simulink model "sampleModel1642"  (R2023a)
settings: Solver=VariableStepAuto  StartTime=0.0  StopTime=10.0  RelTol=1e-3
libraries: hdlsllib x3, simulink x2
settings Model: Creator=user1  LastModifiedBy=user1

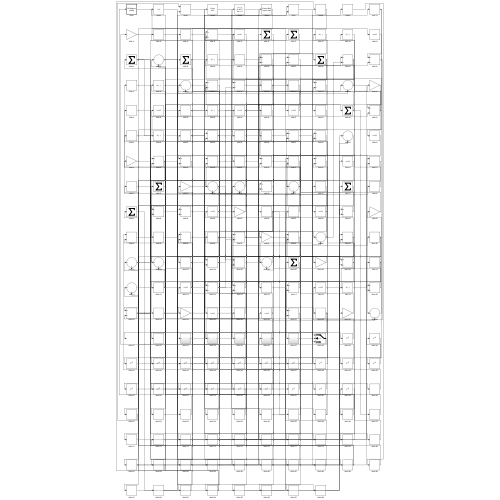
[thumbnail: Simulink's stored preview of the top-level diagram]
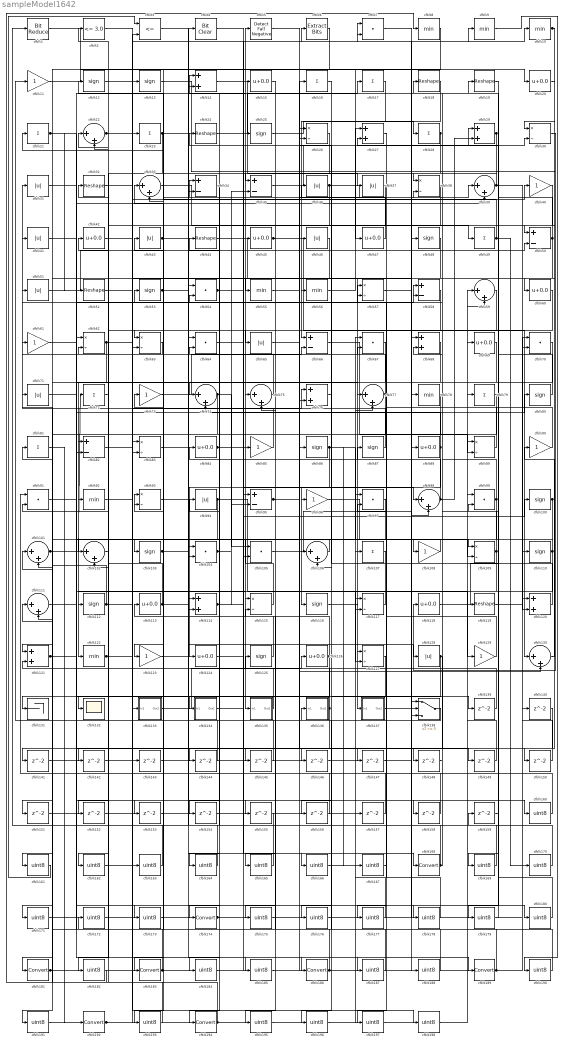
== system sampleModel1642 ==
  cfblk1 : hdlsllib/Logic and Bit Operations/Bit Reduce  mode=AND
  cfblk{8..10,55..56,78,92,122} (8 alike) : MinMax
  cfblk{12..13,25,48,53,80,86..87,100,103,110,112,116,125} (14 alike) : Signum
  cfblk{22,33,39,59,74..75,77,98,101..102,106,111,130} (13 alike) : Sum  Inputs=|++
  cfblk{7,54,64,67,70,91,97,99,104..105} (10 alike) : DotProduct  OutDataTypeStr=Inherit: Inherit via internal rule
  cfblk{16..17,21,23,28,49,72,79,81,107} (10 alike) : Sum  Inputs=+
  cfblk{11,40,61,73,85,90,96,108,123,129} (10 alike) : Gain
  cfblk{26,30,38,57,62..63,83,89,93,109,115,117,127} (13 alike) : Product  Inputs=*/  RndMeth=Zero  SaturateOnIntegerOverflow=on
  cfblk{15,20,42,45,47,60,69,84,88,113,118,124,126} (13 alike) : Bias  Bias=0.0  SaturateOnIntegerOverflow=off
  cfblk{14,27,29,68,76,114,120..121} (8 alike) : Sum
  cfblk{18..19,24,32,44,52,119} (7 alike) : Reshape
  cfblk{31,36..37,41,43,46,51,65,71,94,128} (11 alike) : Abs  SaturateOnIntegerOverflow=off
  cfblk131 : Terminator
  cfblk132 : Scope
  cfblk133 : Subsystem
      settings: LibrarySourceBlock=|
      | hdlsllib/Ports &
      | Subsystems/Subsystem
  cfblk134 : Subsystem
      settings: LibrarySourceBlock=|
      | hdlsllib/Ports &
      | Subsystems/Subsystem
  cfblk135 : Subsystem
      settings: LibrarySourceBlock=|
      | hdlsllib/Ports &
      | Subsystems/Subsystem
  cfblk136 : Subsystem
      settings: LibrarySourceBlock=|
      | hdlsllib/Ports &
      | Subsystems/Subsystem
  cfblk137 : Subsystem
      settings: LibrarySourceBlock=|
      | hdlsllib/Ports &
      | Subsystems/Subsystem
  cfblk138 : Switch  SaturateOnIntegerOverflow=off  InputSameDT=off
  cfblk{139..159} (21 alike) : Delay  SampleTime=1
  cfblk{160..167,169..173,175..180,182,184..185,187..188,190..191,193,195..198} (31 alike) : DataTypeConversion  OutDataTypeStr=uint8  SaturateOnIntegerOverflow=off  RndMeth=Floor
  cfblk{168,174,181,183,186,189,192,194} (8 alike) : DataTypeConversion  SaturateOnIntegerOverflow=off  RndMeth=Floor
  cfblk2 : hdlsllib/Logic and Bit Operations/Compare To Constant  relop=<=  const=3.0  OutDataTypeStr=boolean
  cfblk3 : RelationalOperator  Operator=<=  OutDataTypeStr=boolean  InputSameDT=off
  cfblk{34..35,50,58,66,82,95} (7 alike) : Sum  Inputs=+-
  cfblk4 : simulink/Logic and Bit Operations/Bit Clear  iBit=0
      settings: LibrarySourceBlock=|
      | hdlsllib/Logic and Bit
      | Operations/Bit Clear
  cfblk5 : hdlsllib/Logic and Bit Operations/Detect Fall Negative  vinit=0  OutDataTypeStr=boolean
  cfblk6 : simulink/Logic and Bit Operations/Extract Bits  bitsToExtract=Upper half  numBits=8  bitIdxRange=[0 7]  outScalingMode=Preserve fixed-point scaling
      settings: LibrarySourceBlock=|
      | hdlsllib/Logic and Bit
      | Operations/Extract Bits
  wires:
  cfblk68/1 -> cfblk122/1
  cfblk24/1 -> cfblk17/1
  cfblk109/1 -> cfblk51/1, cfblk193/1
  cfblk118/1 -> cfblk63/1
  cfblk11/1 -> cfblk20/1
  cfblk63/1 -> cfblk31/1
  cfblk101/1 -> cfblk72/1, cfblk80/1
  cfblk8/1 -> cfblk181/1
  cfblk13/1 -> cfblk50/1
  cfblk88/1 -> cfblk124/1, cfblk74/2
  cfblk17/1 -> cfblk66/1
  cfblk120/1 -> cfblk24/1
  cfblk5/1 -> cfblk86/1
  cfblk133/1(Out1) -> cfblk126/1
  cfblk47/1 -> cfblk12/1
  cfblk135/1(Out1) -> cfblk22/1
  cfblk45/1 -> cfblk130/1, cfblk30/2
  cfblk33/1 -> cfblk49/1
  cfblk25/1 -> cfblk28/1
  cfblk83/1 -> cfblk189/1
  cfblk28/1 -> cfblk38/1, cfblk65/1
  cfblk36/1 -> cfblk38/2, cfblk75/2
  cfblk30/1 -> cfblk118/1
  cfblk64/1 -> cfblk168/1
  cfblk82/1 -> cfblk23/1
  cfblk23/1 -> cfblk128/1, cfblk132/1
  cfblk48/1 -> cfblk137/1(In1)
  cfblk86/1 -> cfblk116/1, cfblk108/1, cfblk134/1(In1), cfblk167/1
  cfblk126/1 -> cfblk113/1, cfblk191/1
  cfblk115/1 -> cfblk5/1
  cfblk93/1 -> cfblk4/1
  cfblk14/1 -> cfblk37/1
  cfblk136/1(Out1) -> cfblk93/1, cfblk154/1
  cfblk50/1 -> cfblk14/2, cfblk27/2, cfblk195/1
  cfblk35/1 -> cfblk29/1
  cfblk100/1 -> cfblk135/1(In1), cfblk102/2
  cfblk16/1 -> cfblk96/1
  cfblk69/1 -> cfblk101/2
  cfblk116/1 -> cfblk127/1
  cfblk54/1 -> cfblk158/1, cfblk184/1
  cfblk107/1 -> cfblk174/1
  cfblk39/1 -> cfblk120/2, cfblk35/1
  cfblk81/1 -> cfblk192/1
  cfblk78/1 -> cfblk92/1
  cfblk117/1 -> cfblk114/1
  cfblk51/1 -> cfblk13/1
  cfblk134/1(Out1) -> cfblk85/1
  cfblk138/1 -> cfblk11/1
  cfblk42/1 -> cfblk40/1
  cfblk108/1 -> cfblk103/1
  cfblk77/1 -> cfblk121/1, cfblk36/1, cfblk57/2
  cfblk119/1 -> cfblk110/1
  cfblk73/1 -> cfblk66/2
  cfblk89/1 -> cfblk53/1
  cfblk18/1 -> cfblk46/1
  cfblk96/1 -> cfblk109/1
  cfblk84/1 -> cfblk14/1, cfblk7/2
  cfblk103/1 -> cfblk123/1, cfblk166/1
  cfblk53/1 -> cfblk55/1, cfblk178/1
  cfblk44/1 -> cfblk138/1
  cfblk56/1 -> cfblk27/1
  cfblk71/1 -> cfblk115/1
  cfblk66/1 -> cfblk89/2
  cfblk75/1 -> cfblk44/1
  cfblk26/1 -> cfblk183/1
  cfblk110/1 -> cfblk127/2, cfblk104/1, cfblk162/1
  cfblk92/1 -> cfblk75/1
  cfblk52/1 -> cfblk50/2
  cfblk98/1 -> cfblk84/1, cfblk29/2
  cfblk122/1 -> cfblk9/1, cfblk155/1
  cfblk4/1 -> cfblk98/1
  cfblk121/1 -> cfblk15/1, cfblk138/2, cfblk39/2, cfblk173/1
  cfblk105/1 -> cfblk10/1
  cfblk123/1 -> cfblk76/1
  cfblk7/1 -> cfblk48/1
  cfblk94/1 -> cfblk129/1, cfblk104/2, cfblk35/2
  cfblk46/1 -> cfblk131/1
  cfblk128/1 -> cfblk147/1, cfblk148/1
  cfblk106/1 -> cfblk102/1
  cfblk1/1 -> cfblk47/1
  cfblk60/1 -> cfblk106/1
  cfblk99/1 -> cfblk68/2, cfblk112/1, cfblk141/1
  cfblk80/1 -> cfblk19/1
  cfblk41/1 -> cfblk74/1
  cfblk38/1 -> cfblk82/1
  cfblk111/1 -> cfblk186/1
  cfblk85/1 -> cfblk41/1
  cfblk114/1 -> cfblk100/1, cfblk45/1
  cfblk91/1 -> cfblk58/1
  cfblk10/1 -> cfblk60/1, cfblk30/1
  cfblk112/1 -> cfblk71/1, cfblk180/1
  cfblk6/1 -> cfblk33/2
  cfblk57/1 -> cfblk88/1
  cfblk130/1 -> cfblk90/1
  cfblk43/1 -> cfblk6/1, cfblk7/1
  cfblk72/1 -> cfblk32/1
  cfblk76/1 -> cfblk106/2
  cfblk104/1 -> cfblk95/2, cfblk164/1
  cfblk29/1 -> cfblk138/3, cfblk177/1
  cfblk95/1 -> cfblk130/2, cfblk57/1
  cfblk12/1 -> cfblk77/1
  cfblk74/1 -> cfblk105/1, cfblk151/1
  cfblk125/1 -> cfblk34/1
  cfblk87/1 -> cfblk34/2
  cfblk113/1 -> cfblk91/2, cfblk139/1
  cfblk79/1 -> cfblk194/1
  cfblk90/1 -> cfblk61/1
  cfblk62/1 -> cfblk82/2, cfblk198/1
  cfblk65/1 -> cfblk39/1
  cfblk129/1 -> cfblk87/1
  cfblk21/1 -> cfblk109/2, cfblk52/1, cfblk185/1
  cfblk124/1 -> cfblk25/1
  cfblk49/1 -> cfblk21/1, cfblk170/1
  cfblk22/1 -> cfblk133/1(In1), cfblk56/1
  cfblk139/1 -> cfblk121/2
  cfblk141/1 -> cfblk117/2
  cfblk37/1 -> cfblk142/1
  cfblk142/1 -> cfblk22/2
  cfblk32/1 -> cfblk143/1
  cfblk143/1 -> cfblk114/2
  cfblk34/1 -> cfblk144/1
  cfblk144/1 -> cfblk93/2
  cfblk40/1 -> cfblk145/1
  cfblk145/1 -> cfblk101/1
  cfblk61/1 -> cfblk146/1
  cfblk146/1 -> cfblk68/1
  cfblk147/1 -> cfblk98/2
  cfblk148/1 -> cfblk58/2
  cfblk55/1 -> cfblk149/1
  cfblk149/1 -> cfblk89/1
  cfblk20/1 -> cfblk150/1
  cfblk150/1 -> cfblk120/1
  cfblk151/1 -> cfblk95/1
  cfblk102/1 -> cfblk152/1
  cfblk31/1 -> cfblk153/1
  cfblk153/1 -> cfblk33/1
  cfblk154/1 -> cfblk77/2
  cfblk155/1 -> cfblk1/1
  cfblk127/1 -> cfblk156/1
  cfblk156/1 -> cfblk115/2
  cfblk157/1 -> cfblk54/2
  cfblk158/1 -> cfblk91/1
  cfblk3/1 -> cfblk160/1
  cfblk160/1 -> cfblk43/1
  cfblk140/1 -> cfblk161/1
  cfblk161/1 -> cfblk3/1
  cfblk162/1 -> cfblk3/2
  cfblk2/1 -> cfblk163/1
  cfblk163/1 -> cfblk42/1
  cfblk164/1 -> cfblk2/1
  cfblk67/1 -> cfblk165/1
  cfblk165/1 -> cfblk54/1
  cfblk166/1 -> cfblk67/1
  cfblk167/1 -> cfblk67/2
  cfblk168/1 -> cfblk18/1, cfblk94/1
  cfblk19/1 -> cfblk169/1
  cfblk169/1 -> cfblk64/1
  cfblk170/1 -> cfblk64/2
  cfblk70/1 -> cfblk171/1
  cfblk171/1 -> cfblk76/2
  cfblk172/1 -> cfblk70/1
  cfblk173/1 -> cfblk70/2
  cfblk174/1 -> cfblk16/1, cfblk119/1
  cfblk15/1 -> cfblk175/1
  cfblk175/1 -> cfblk107/1
  cfblk97/1 -> cfblk176/1
  cfblk176/1 -> cfblk78/1
  cfblk177/1 -> cfblk97/1
  cfblk178/1 -> cfblk97/2
  cfblk159/1 -> cfblk179/1
  cfblk179/1 -> cfblk99/2
  cfblk180/1 -> cfblk159/1
  cfblk181/1 -> cfblk140/1, cfblk99/1
  cfblk58/1 -> cfblk182/1
  cfblk182/1 -> cfblk8/1
  cfblk183/1 -> cfblk105/2, cfblk62/1
  cfblk184/1 -> cfblk26/1
  cfblk185/1 -> cfblk26/2
  cfblk186/1 -> cfblk125/1, cfblk69/1
  cfblk152/1 -> cfblk187/1
  cfblk187/1 -> cfblk111/1
  cfblk137/1(Out1) -> cfblk188/1
  cfblk188/1 -> cfblk111/2
  cfblk189/1 -> cfblk73/1, cfblk136/1(In1)
  cfblk9/1 -> cfblk190/1
  cfblk190/1 -> cfblk83/1
  cfblk191/1 -> cfblk83/2
  cfblk192/1 -> cfblk63/2, cfblk117/1
  cfblk193/1 -> cfblk81/1
  cfblk194/1 -> cfblk172/1, cfblk62/2
  cfblk195/1 -> cfblk79/1
  cfblk59/1 -> cfblk196/1
  cfblk196/1 -> cfblk157/1
  cfblk27/1 -> cfblk197/1
  cfblk197/1 -> cfblk59/1
  cfblk198/1 -> cfblk59/2

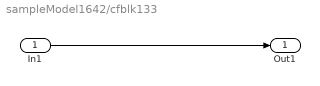
== system sampleModel1642/cfblk133 ==
  In1 : Inport
  Out1 : Outport
  wires:
  In1/1 -> Out1/1

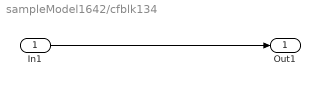
== system sampleModel1642/cfblk134 ==
  In1 : Inport
  Out1 : Outport
  wires:
  In1/1 -> Out1/1

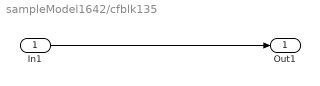
== system sampleModel1642/cfblk135 ==
  In1 : Inport
  Out1 : Outport
  wires:
  In1/1 -> Out1/1

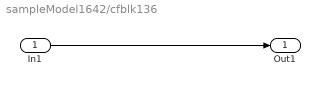
== system sampleModel1642/cfblk136 ==
  In1 : Inport
  Out1 : Outport
  wires:
  In1/1 -> Out1/1

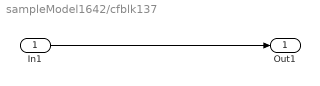
== system sampleModel1642/cfblk137 ==
  In1 : Inport
  Out1 : Outport
  wires:
  In1/1 -> Out1/1
